simulink model "lab1_system6"  (R2024a)
settings: Solver=VariableStepAuto  StartTime=0.0  StopTime=10.0  RelTol=1e-3
settings Model: Creator=alexivanov  LastModifiedBy=alexivanov

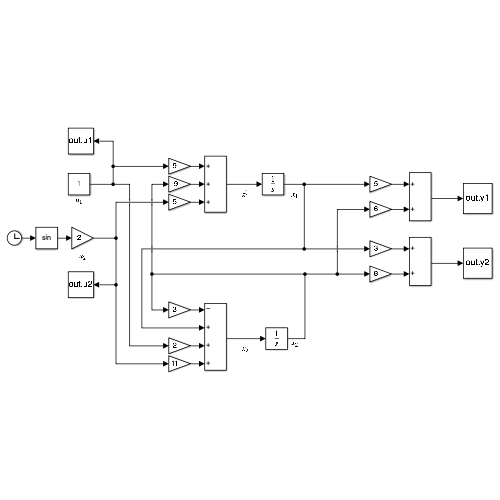
[thumbnail: Simulink's stored preview of the top-level diagram]
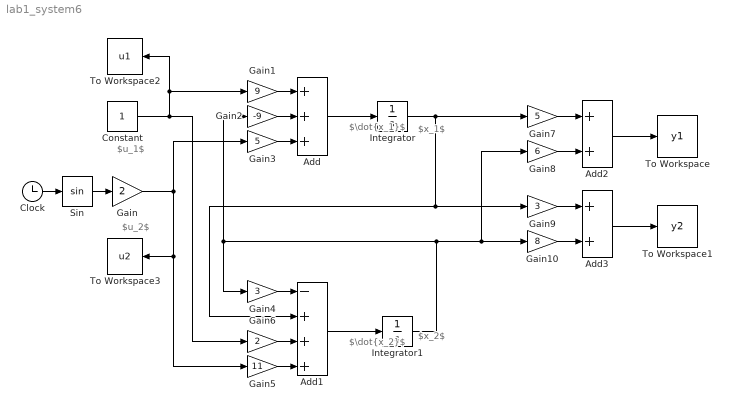
== system lab1_system6 ==
  note: $u_2$
  note: $u_1$
  note: $x_1$
  note: $x_2$
  note: $\dot{x_1}$
  note: $\dot{x_2}$
  Add : Sum  Inputs=+++
  Add1 : Sum  Inputs=-+++
  Add2 : Sum
  Add3 : Sum
  Clock : Clock
  Constant : Constant  SampleTime=0
  Gain : Gain  Gain=2
  Gain1 : Gain  Gain=9
  Gain10 : Gain  Gain=8
  Gain2 : Gain  Gain=-9
  Gain3 : Gain  Gain=5
  Gain4 : Gain  Gain=3
  Gain5 : Gain  Gain=11
  Gain6 : Gain  Gain=2
  Gain7 : Gain  Gain=5
  Gain8 : Gain  Gain=6
  Gain9 : Gain  Gain=3
  Integrator : Integrator
  Integrator1 : Integrator
  Sin : Trigonometry
  To Workspace : ToWorkspace  VariableName=y1  SaveFormat=Timeseries  SampleTime=-1
  To Workspace1 : ToWorkspace  VariableName=y2  SaveFormat=Timeseries  SampleTime=-1
  To Workspace2 : ToWorkspace  VariableName=u1  SaveFormat=Timeseries  SampleTime=-1
  To Workspace3 : ToWorkspace  VariableName=u2  SaveFormat=Timeseries  SampleTime=-1
  wires:
  Clock/1 -> Sin/1
  Sin/1 -> Gain/1
  Gain/1 -> Gain3/1, Gain5/1, To Workspace3/1
  Constant/1 -> Gain6/1, Gain1/1, To Workspace2/1
  Gain1/1 -> Add/1
  Gain3/1 -> Add/3
  Gain2/1 -> Add/2
  Add/1 -> Integrator/1
  Integrator1/1 -> Gain10/1, Gain8/1, Gain4/1, Gain2/1
  Integrator/1 -> Gain7/1, Gain9/1, Add1/2
  Gain6/1 -> Add1/3
  Gain4/1 -> Add1/1
  Add1/1 -> Integrator1/1
  Gain5/1 -> Add1/4
  Add2/1 -> To Workspace/1
  Gain7/1 -> Add2/1
  Gain8/1 -> Add2/2
  Gain9/1 -> Add3/1
  Gain10/1 -> Add3/2
  Add3/1 -> To Workspace1/1
